simulink model "Roadsense_VehicleDynamics"  (R2025b)
settings: Solver=FixedStepDiscrete  StartTime=0.0  StopTime=1.0  FixedStep=RsTsBase  RelTol=1e-3
undefined symbols (not defined in the file or in its folder): RsTsControl, RsVehicleMass
settings Model: DataDictionary=Roadsense_Data.sldd  Creator=ragur  LastModifiedBy=ragur

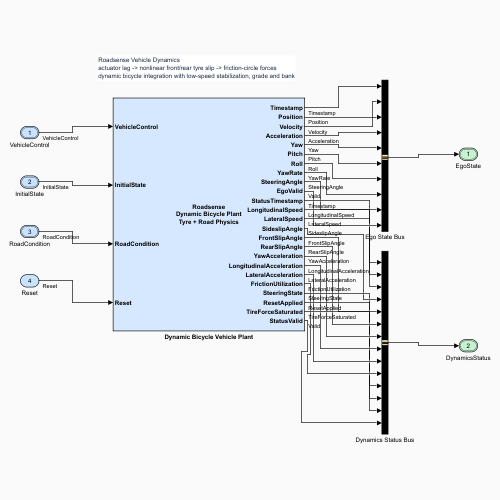
[thumbnail: Simulink's stored preview of the top-level diagram]
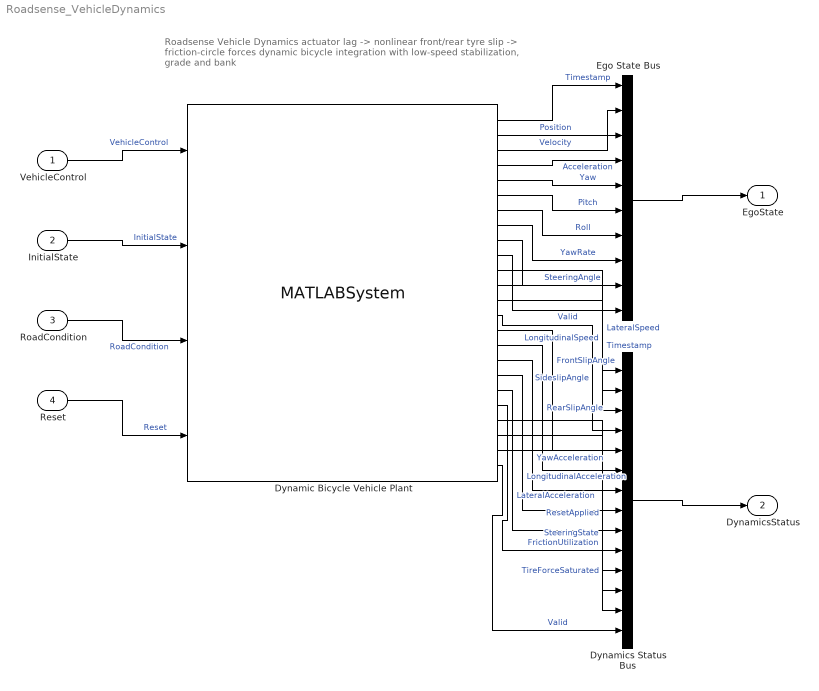
== system Roadsense_VehicleDynamics ==
  note: Roadsense Vehicle Dynamics
      | actuator lag -> nonlinear front/rear tyre slip -> friction-circle forces
      | dynamic bicycle integration with low-speed stabilization, grade and bank
  VehicleControl : Inport  OutDataTypeStr=Bus: RsVehicleControlBus  PortDimensions=1  SampleTime=RsTsControl
  InitialState : Inport  Port=2  OutDataTypeStr=Bus: RsEgoStateBus  PortDimensions=1  SampleTime=RsTsControl
  RoadCondition : Inport  Port=3  OutDataTypeStr=Bus: RsRoadConditionBus  PortDimensions=1  SampleTime=RsTsControl
  Reset : Inport  Port=4  OutDataTypeStr=boolean  PortDimensions=1  SampleTime=RsTsControl
  Dynamic Bicycle Vehicle Plant : MATLABSystem  System=RoadsenseVehicleDynamicsSystem  SampleTime=RsTsControl  Mass=RsVehicleMass  YawInertia=RsVehicleYawInertia  FrontAxleDistance=RsVehicleFrontAxleDistance  RearAxleDistance=RsVehicleRearAxleDistance  FrontCorneringStiffness=RsVehicleFrontCorneringStiffness  RearCorneringStiffness=RsVehicleRearCorneringStiffness  SteeringTimeConstant=RsVehicleSteeringTimeConstant  AccelerationTimeConstant=RsVehicleAccelerationTimeConstant  MaximumSteering=RsControllerMaximumSteering  MaximumSteeringRate=RsVehicleMaximumSteeringRate  MaximumAcceleration=RsControllerMaximumAcceleration  MaximumDeceleration=RsControllerMaximumDeceleration  MaximumJerk=RsVehicleMaximumJerk  LowSpeedThreshold=RsVehicleLowSpeedThreshold  MaximumSpeed=RsVehicleMaximumSpeed  Gravity=single(9.8100004196167)  SimulateUsing=Code generation
      mask Type: RoadsenseVehicleDynamicsSystem
  Dynamics Status Bus : BusCreator  Inputs=14  OutDataTypeStr=Bus: RsVehicleDynamicsStatusBus
  Ego State Bus : BusCreator  Inputs=10  OutDataTypeStr=Bus: RsEgoStateBus
  EgoState : Outport  OutDataTypeStr=Bus: RsEgoStateBus
  DynamicsStatus : Outport  Port=2  OutDataTypeStr=Bus: RsVehicleDynamicsStatusBus
  wires:
  VehicleControl/1 -> Dynamic Bicycle Vehicle Plant/1  "VehicleControl"
  InitialState/1 -> Dynamic Bicycle Vehicle Plant/2  "InitialState"
  RoadCondition/1 -> Dynamic Bicycle Vehicle Plant/3  "RoadCondition"
  Reset/1 -> Dynamic Bicycle Vehicle Plant/4  "Reset"
  Dynamic Bicycle Vehicle Plant/1 -> Ego State Bus/1  "Timestamp"
  Dynamic Bicycle Vehicle Plant/2 -> Ego State Bus/2  "Position"
  Dynamic Bicycle Vehicle Plant/3 -> Ego State Bus/3  "Velocity"
  Dynamic Bicycle Vehicle Plant/4 -> Ego State Bus/4  "Acceleration"
  Dynamic Bicycle Vehicle Plant/5 -> Ego State Bus/5  "Yaw"
  Dynamic Bicycle Vehicle Plant/6 -> Ego State Bus/6  "Pitch"
  Dynamic Bicycle Vehicle Plant/7 -> Ego State Bus/7  "Roll"
  Dynamic Bicycle Vehicle Plant/8 -> Ego State Bus/8  "YawRate"
  Dynamic Bicycle Vehicle Plant/9 -> Ego State Bus/9  "SteeringAngle"
  Dynamic Bicycle Vehicle Plant/10 -> Ego State Bus/10  "Valid"
  Dynamic Bicycle Vehicle Plant/11 -> Dynamics Status Bus/1  "Timestamp"
  Dynamic Bicycle Vehicle Plant/12 -> Dynamics Status Bus/2  "LongitudinalSpeed"
  Dynamic Bicycle Vehicle Plant/13 -> Dynamics Status Bus/3  "LateralSpeed"
  Dynamic Bicycle Vehicle Plant/14 -> Dynamics Status Bus/4  "SideslipAngle"
  Dynamic Bicycle Vehicle Plant/15 -> Dynamics Status Bus/5  "FrontSlipAngle"
  Dynamic Bicycle Vehicle Plant/16 -> Dynamics Status Bus/6  "RearSlipAngle"
  Dynamic Bicycle Vehicle Plant/17 -> Dynamics Status Bus/7  "YawAcceleration"
  Dynamic Bicycle Vehicle Plant/18 -> Dynamics Status Bus/8  "LongitudinalAcceleration"
  Dynamic Bicycle Vehicle Plant/19 -> Dynamics Status Bus/9  "LateralAcceleration"
  Dynamic Bicycle Vehicle Plant/20 -> Dynamics Status Bus/10  "FrictionUtilization"
  Dynamic Bicycle Vehicle Plant/21 -> Dynamics Status Bus/11  "SteeringState"
  Dynamic Bicycle Vehicle Plant/22 -> Dynamics Status Bus/12  "ResetApplied"
  Dynamic Bicycle Vehicle Plant/23 -> Dynamics Status Bus/13  "TireForceSaturated"
  Dynamic Bicycle Vehicle Plant/24 -> Dynamics Status Bus/14  "Valid"
  Ego State Bus/1 -> EgoState/1
  Dynamics Status Bus/1 -> DynamicsStatus/1
